simulink model "comparasion"  (R2023a)
settings: Solver=VariableStepAuto  StartTime=0.0  StopTime=3  RelTol=1e-3
values from neighbouring files (symbols this model uses):
  A = [a11 a21 a12 a22]    [calc_A.m]    (also in modelo.m = [a11 a12)
  Ad = [-1/t_beta 0 ... (first row only)    [calc_KMax.m]    (also in calc_Kmin.m; modelo.m)
  B = [b11 b21 b12 b22]    [calc_B.m]    (also in calc_inv_B.m = [b11 b12; b21 b22]; modelo.m = [b11 b12)
  C = [1 0 ... (first row only)    [modelo.m]
  D = [0 0;0 0]    [modelo.m]
  E = [e1 e2]    [calc_E.m]    (also in modelo.m = [e1)
  Ed = [k_beta/t_beta ... (first row only)    [calc_KMax.m]    (also in calc_Kmin.m; modelo.m)
  k1 = L_1(A,B,B2,C3,D32,D31,lambda)    [modelo.m]
  k2 = H_2_gain(A,B,B2,C2,D22)    [modelo.m]
  kH2Hinf = H_2_H_inf(A,B,B2,C2,D22,C1,D12,D11,a,b)    [modelo.m]
  kinf = H_inf(A,B,B2,C1,D12,D11)    [modelo.m]
  kLQ = LQ(Cz,Dzu,A,B,0)    [modelo.m]
  kLQR = LQ_R(Cz,Dzu,A,B,alpha,theta,r)    [modelo.m]
  x0 = [0, 0]    [modelo.m]
undefined symbols (not defined in the file or in its folder): sigbuilder_block
settings Model: Creator=Ferna  LastModifiedBy=Ferna

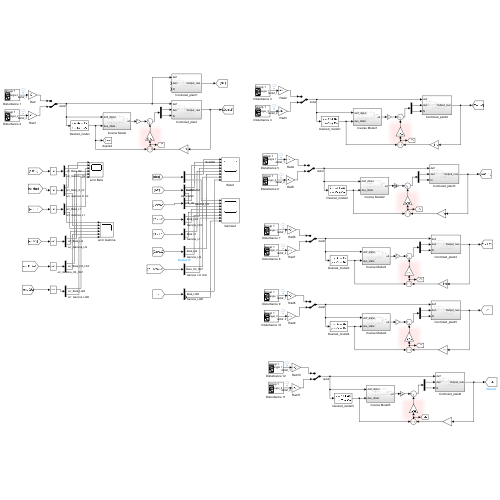
[thumbnail: Simulink's stored preview of the top-level diagram]
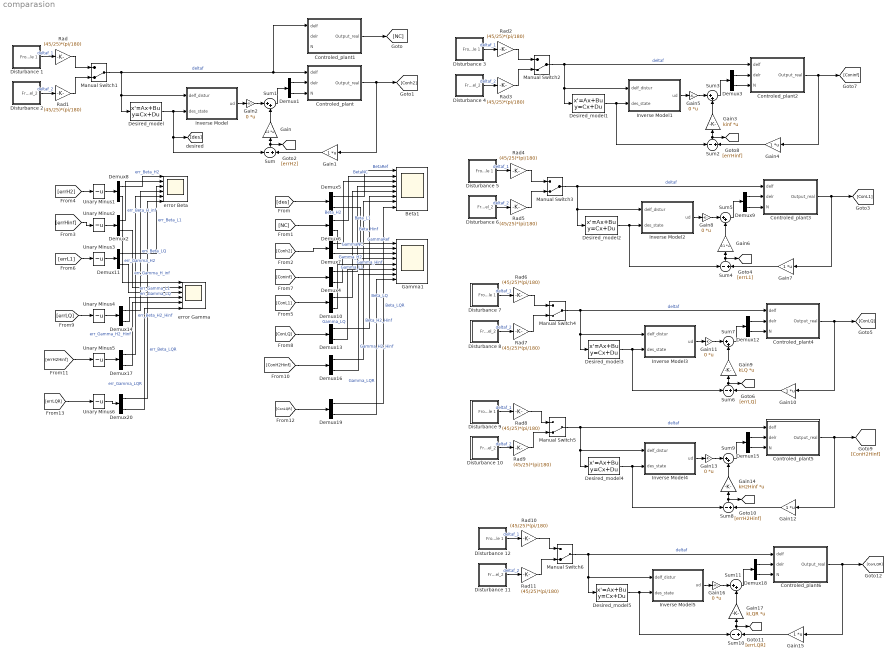
== system comparasion ==
  Beta1 : Scope  NumInputPorts=8
  Controled_plant : Subsystem
  Controled_plant1 : Subsystem
  Controled_plant2 : Subsystem
  Controled_plant3 : Subsystem
  Controled_plant4 : Subsystem
  Controled_plant5 : Subsystem
  Controled_plant6 : Subsystem
  Demux{1..20} (20 alike) : Demux  Outputs=2
  Desired_model{,1..5} (6 alike) : StateSpace  A=Ad  B=Ed  C=[1,0;0,1]  D=zeros(2,1)  InitialCondition=0
  Disturbance 1 : Subsystem  Tag=STV Subsys  LoadFcn=sigbuilder_block('load');  StartFcn=sigbuilder_block('start');  StopFcn=sigbuilder_block('stop');  ClipboardFcn=sigbuilder_block('clipboard');  mask(Sigbuilder block){tuvar=[0:10]}
      mask help: Simulink:masks:SigbuilderBlock_MD
      mask init:
      | if ~strcmp(get_param(bdroot(gcbh),'SimulationStatus'),'stopped') tuvar = sigbuilder_block('maskInit'); end
      settings: CopyFcn=sigbuilder_block('copy');  DeleteFcn=sigbuilder_block('delete');  ModelCloseFcn=sigbuilder_block('modelClose');  PreSaveFcn=sigbuilder_block('preSave');  PauseFcn=sigbuilder_block('pause');  ContinueFcn=sigbuilder_block('continue');  NameChangeFcn=sigbuilder_block('namechange');  OpenFcn=sigbuilder_block('open',[265.8 141.6 550.8 400.2 ]);  CloseFcn=sigbuilder_block('close');
      mask Display: plot(0, 0, 100, 100,[2, 2, 32, 32, 2], [68, 8, 8, 68, 68],[32, 2], [38, 38], [32, 19, 2],[53, 60, 44], [32, 17, 17, 2],[16, 16, 31, 31]);txt = getActiveGroup(gcbh);text(2, 100, txt,'verticalAlignment', 'top');
  Disturbance 10 : Subsystem  Tag=STV Subsys  LoadFcn=sigbuilder_block('load');  StartFcn=sigbuilder_block('start');  StopFcn=sigbuilder_block('stop');  ClipboardFcn=sigbuilder_block('clipboard');  mask(Sigbuilder block){tuvar=[0:10]}
      mask help: Simulink:masks:SigbuilderBlock_MD
      mask init:
      | if ~strcmp(get_param(bdroot(gcbh),'SimulationStatus'),'stopped') tuvar = sigbuilder_block('maskInit'); end
      settings: CopyFcn=sigbuilder_block('copy');  DeleteFcn=sigbuilder_block('delete');  ModelCloseFcn=sigbuilder_block('modelClose');  PreSaveFcn=sigbuilder_block('preSave');  PauseFcn=sigbuilder_block('pause');  ContinueFcn=sigbuilder_block('continue');  NameChangeFcn=sigbuilder_block('namechange');  OpenFcn=sigbuilder_block('open',[265.8 141.6 550.8 400.2 ]);  CloseFcn=sigbuilder_block('close');
      mask Display: plot(0, 0, 100, 100,[2, 2, 32, 32, 2], [68, 8, 8, 68, 68],[32, 2], [38, 38], [32, 19, 2],[53, 60, 44], [32, 17, 17, 2],[16, 16, 31, 31]);txt = getActiveGroup(gcbh);text(2, 100, txt,'verticalAlignment', 'top');
  Disturbance 11 : Subsystem  Tag=STV Subsys  LoadFcn=sigbuilder_block('load');  StartFcn=sigbuilder_block('start');  StopFcn=sigbuilder_block('stop');  ClipboardFcn=sigbuilder_block('clipboard');  mask(Sigbuilder block){tuvar=[0:10]}
      mask help: Simulink:masks:SigbuilderBlock_MD
      mask init:
      | if ~strcmp(get_param(bdroot(gcbh),'SimulationStatus'),'stopped') tuvar = sigbuilder_block('maskInit'); end
      settings: CopyFcn=sigbuilder_block('copy');  DeleteFcn=sigbuilder_block('delete');  ModelCloseFcn=sigbuilder_block('modelClose');  PreSaveFcn=sigbuilder_block('preSave');  PauseFcn=sigbuilder_block('pause');  ContinueFcn=sigbuilder_block('continue');  NameChangeFcn=sigbuilder_block('namechange');  OpenFcn=sigbuilder_block('open',[265.8 141.6 550.8 400.2 ]);  CloseFcn=sigbuilder_block('close');
      mask Display: plot(0, 0, 100, 100,[2, 2, 32, 32, 2], [68, 8, 8, 68, 68],[32, 2], [38, 38], [32, 19, 2],[53, 60, 44], [32, 17, 17, 2],[16, 16, 31, 31]);txt = getActiveGroup(gcbh);text(2, 100, txt,'verticalAlignment', 'top');
  Disturbance 12 : Subsystem  Tag=STV Subsys  LoadFcn=sigbuilder_block('load');  StartFcn=sigbuilder_block('start');  StopFcn=sigbuilder_block('stop');  ClipboardFcn=sigbuilder_block('clipboard');  mask(Sigbuilder block){tuvar=[0:10]}
      mask help: Simulink:masks:SigbuilderBlock_MD
      mask init:
      | if ~strcmp(get_param(bdroot(gcbh),'SimulationStatus'),'stopped') tuvar = sigbuilder_block('maskInit'); end
      settings: CopyFcn=sigbuilder_block('copy');  DeleteFcn=sigbuilder_block('delete');  ModelCloseFcn=sigbuilder_block('modelClose');  PreSaveFcn=sigbuilder_block('preSave');  PauseFcn=sigbuilder_block('pause');  ContinueFcn=sigbuilder_block('continue');  NameChangeFcn=sigbuilder_block('namechange');  OpenFcn=sigbuilder_block('open',[265.8 141.6 550.8 400.2 ]);  CloseFcn=sigbuilder_block('close');
      mask Display: plot(0, 0, 100, 100,[2, 2, 32, 32, 2], [68, 8, 8, 68, 68],[32, 2], [38, 38], [32, 19, 2],[53, 60, 44], [32, 17, 17, 2],[16, 16, 31, 31]);txt = getActiveGroup(gcbh);text(2, 100, txt,'verticalAlignment', 'top');
  Disturbance 2 : Subsystem  Tag=STV Subsys  LoadFcn=sigbuilder_block('load');  StartFcn=sigbuilder_block('start');  StopFcn=sigbuilder_block('stop');  ClipboardFcn=sigbuilder_block('clipboard');  mask(Sigbuilder block){tuvar=[0:10]}
      mask help: Simulink:masks:SigbuilderBlock_MD
      mask init:
      | if ~strcmp(get_param(bdroot(gcbh),'SimulationStatus'),'stopped') tuvar = sigbuilder_block('maskInit'); end
      settings: CopyFcn=sigbuilder_block('copy');  DeleteFcn=sigbuilder_block('delete');  ModelCloseFcn=sigbuilder_block('modelClose');  PreSaveFcn=sigbuilder_block('preSave');  PauseFcn=sigbuilder_block('pause');  ContinueFcn=sigbuilder_block('continue');  NameChangeFcn=sigbuilder_block('namechange');  OpenFcn=sigbuilder_block('open',[265.8 141.6 550.8 400.2 ]);  CloseFcn=sigbuilder_block('close');
      mask Display: plot(0, 0, 100, 100,[2, 2, 32, 32, 2], [68, 8, 8, 68, 68],[32, 2], [38, 38], [32, 19, 2],[53, 60, 44], [32, 17, 17, 2],[16, 16, 31, 31]);txt = getActiveGroup(gcbh);text(2, 100, txt,'verticalAlignment', 'top');
  Disturbance 3 : Subsystem  Tag=STV Subsys  LoadFcn=sigbuilder_block('load');  StartFcn=sigbuilder_block('start');  StopFcn=sigbuilder_block('stop');  ClipboardFcn=sigbuilder_block('clipboard');  mask(Sigbuilder block){tuvar=[0:10]}
      mask help: Simulink:masks:SigbuilderBlock_MD
      mask init:
      | if ~strcmp(get_param(bdroot(gcbh),'SimulationStatus'),'stopped') tuvar = sigbuilder_block('maskInit'); end
      settings: CopyFcn=sigbuilder_block('copy');  DeleteFcn=sigbuilder_block('delete');  ModelCloseFcn=sigbuilder_block('modelClose');  PreSaveFcn=sigbuilder_block('preSave');  PauseFcn=sigbuilder_block('pause');  ContinueFcn=sigbuilder_block('continue');  NameChangeFcn=sigbuilder_block('namechange');  OpenFcn=sigbuilder_block('open',[265.8 141.6 550.8 400.2 ]);  CloseFcn=sigbuilder_block('close');
      mask Display: plot(0, 0, 100, 100,[2, 2, 32, 32, 2], [68, 8, 8, 68, 68],[32, 2], [38, 38], [32, 19, 2],[53, 60, 44], [32, 17, 17, 2],[16, 16, 31, 31]);txt = getActiveGroup(gcbh);text(2, 100, txt,'verticalAlignment', 'top');
  Disturbance 4 : Subsystem  Tag=STV Subsys  LoadFcn=sigbuilder_block('load');  StartFcn=sigbuilder_block('start');  StopFcn=sigbuilder_block('stop');  ClipboardFcn=sigbuilder_block('clipboard');  mask(Sigbuilder block){tuvar=[0:10]}
      mask help: Simulink:masks:SigbuilderBlock_MD
      mask init:
      | if ~strcmp(get_param(bdroot(gcbh),'SimulationStatus'),'stopped') tuvar = sigbuilder_block('maskInit'); end
      settings: CopyFcn=sigbuilder_block('copy');  DeleteFcn=sigbuilder_block('delete');  ModelCloseFcn=sigbuilder_block('modelClose');  PreSaveFcn=sigbuilder_block('preSave');  PauseFcn=sigbuilder_block('pause');  ContinueFcn=sigbuilder_block('continue');  NameChangeFcn=sigbuilder_block('namechange');  OpenFcn=sigbuilder_block('open',[265.8 141.6 550.8 400.2 ]);  CloseFcn=sigbuilder_block('close');
      mask Display: plot(0, 0, 100, 100,[2, 2, 32, 32, 2], [68, 8, 8, 68, 68],[32, 2], [38, 38], [32, 19, 2],[53, 60, 44], [32, 17, 17, 2],[16, 16, 31, 31]);txt = getActiveGroup(gcbh);text(2, 100, txt,'verticalAlignment', 'top');
  Disturbance 5 : Subsystem  Tag=STV Subsys  LoadFcn=sigbuilder_block('load');  StartFcn=sigbuilder_block('start');  StopFcn=sigbuilder_block('stop');  ClipboardFcn=sigbuilder_block('clipboard');  mask(Sigbuilder block){tuvar=[0:10]}
      mask help: Simulink:masks:SigbuilderBlock_MD
      mask init:
      | if ~strcmp(get_param(bdroot(gcbh),'SimulationStatus'),'stopped') tuvar = sigbuilder_block('maskInit'); end
      settings: CopyFcn=sigbuilder_block('copy');  DeleteFcn=sigbuilder_block('delete');  ModelCloseFcn=sigbuilder_block('modelClose');  PreSaveFcn=sigbuilder_block('preSave');  PauseFcn=sigbuilder_block('pause');  ContinueFcn=sigbuilder_block('continue');  NameChangeFcn=sigbuilder_block('namechange');  OpenFcn=sigbuilder_block('open',[265.8 141.6 550.8 400.2 ]);  CloseFcn=sigbuilder_block('close');
      mask Display: plot(0, 0, 100, 100,[2, 2, 32, 32, 2], [68, 8, 8, 68, 68],[32, 2], [38, 38], [32, 19, 2],[53, 60, 44], [32, 17, 17, 2],[16, 16, 31, 31]);txt = getActiveGroup(gcbh);text(2, 100, txt,'verticalAlignment', 'top');
  Disturbance 6 : Subsystem  Tag=STV Subsys  LoadFcn=sigbuilder_block('load');  StartFcn=sigbuilder_block('start');  StopFcn=sigbuilder_block('stop');  ClipboardFcn=sigbuilder_block('clipboard');  mask(Sigbuilder block){tuvar=[0:10]}
      mask help: Simulink:masks:SigbuilderBlock_MD
      mask init:
      | if ~strcmp(get_param(bdroot(gcbh),'SimulationStatus'),'stopped') tuvar = sigbuilder_block('maskInit'); end
      settings: CopyFcn=sigbuilder_block('copy');  DeleteFcn=sigbuilder_block('delete');  ModelCloseFcn=sigbuilder_block('modelClose');  PreSaveFcn=sigbuilder_block('preSave');  PauseFcn=sigbuilder_block('pause');  ContinueFcn=sigbuilder_block('continue');  NameChangeFcn=sigbuilder_block('namechange');  OpenFcn=sigbuilder_block('open',[265.8 141.6 550.8 400.2 ]);  CloseFcn=sigbuilder_block('close');
      mask Display: plot(0, 0, 100, 100,[2, 2, 32, 32, 2], [68, 8, 8, 68, 68],[32, 2], [38, 38], [32, 19, 2],[53, 60, 44], [32, 17, 17, 2],[16, 16, 31, 31]);txt = getActiveGroup(gcbh);text(2, 100, txt,'verticalAlignment', 'top');
  Disturbance 7 : Subsystem  Tag=STV Subsys  LoadFcn=sigbuilder_block('load');  StartFcn=sigbuilder_block('start');  StopFcn=sigbuilder_block('stop');  ClipboardFcn=sigbuilder_block('clipboard');  mask(Sigbuilder block){tuvar=[0:10]}
      mask help: Simulink:masks:SigbuilderBlock_MD
      mask init:
      | if ~strcmp(get_param(bdroot(gcbh),'SimulationStatus'),'stopped') tuvar = sigbuilder_block('maskInit'); end
      settings: CopyFcn=sigbuilder_block('copy');  DeleteFcn=sigbuilder_block('delete');  ModelCloseFcn=sigbuilder_block('modelClose');  PreSaveFcn=sigbuilder_block('preSave');  PauseFcn=sigbuilder_block('pause');  ContinueFcn=sigbuilder_block('continue');  NameChangeFcn=sigbuilder_block('namechange');  OpenFcn=sigbuilder_block('open',[265.8 141.6 550.8 400.2 ]);  CloseFcn=sigbuilder_block('close');
      mask Display: plot(0, 0, 100, 100,[2, 2, 32, 32, 2], [68, 8, 8, 68, 68],[32, 2], [38, 38], [32, 19, 2],[53, 60, 44], [32, 17, 17, 2],[16, 16, 31, 31]);txt = getActiveGroup(gcbh);text(2, 100, txt,'verticalAlignment', 'top');
  Disturbance 8 : Subsystem  Tag=STV Subsys  LoadFcn=sigbuilder_block('load');  StartFcn=sigbuilder_block('start');  StopFcn=sigbuilder_block('stop');  ClipboardFcn=sigbuilder_block('clipboard');  mask(Sigbuilder block){tuvar=[0:10]}
      mask help: Simulink:masks:SigbuilderBlock_MD
      mask init:
      | if ~strcmp(get_param(bdroot(gcbh),'SimulationStatus'),'stopped') tuvar = sigbuilder_block('maskInit'); end
      settings: CopyFcn=sigbuilder_block('copy');  DeleteFcn=sigbuilder_block('delete');  ModelCloseFcn=sigbuilder_block('modelClose');  PreSaveFcn=sigbuilder_block('preSave');  PauseFcn=sigbuilder_block('pause');  ContinueFcn=sigbuilder_block('continue');  NameChangeFcn=sigbuilder_block('namechange');  OpenFcn=sigbuilder_block('open',[265.8 141.6 550.8 400.2 ]);  CloseFcn=sigbuilder_block('close');
      mask Display: plot(0, 0, 100, 100,[2, 2, 32, 32, 2], [68, 8, 8, 68, 68],[32, 2], [38, 38], [32, 19, 2],[53, 60, 44], [32, 17, 17, 2],[16, 16, 31, 31]);txt = getActiveGroup(gcbh);text(2, 100, txt,'verticalAlignment', 'top');
  Disturbance 9 : Subsystem  Tag=STV Subsys  LoadFcn=sigbuilder_block('load');  StartFcn=sigbuilder_block('start');  StopFcn=sigbuilder_block('stop');  ClipboardFcn=sigbuilder_block('clipboard');  mask(Sigbuilder block){tuvar=[0:10]}
      mask help: Simulink:masks:SigbuilderBlock_MD
      mask init:
      | if ~strcmp(get_param(bdroot(gcbh),'SimulationStatus'),'stopped') tuvar = sigbuilder_block('maskInit'); end
      settings: CopyFcn=sigbuilder_block('copy');  DeleteFcn=sigbuilder_block('delete');  ModelCloseFcn=sigbuilder_block('modelClose');  PreSaveFcn=sigbuilder_block('preSave');  PauseFcn=sigbuilder_block('pause');  ContinueFcn=sigbuilder_block('continue');  NameChangeFcn=sigbuilder_block('namechange');  OpenFcn=sigbuilder_block('open',[265.8 141.6 550.8 400.2 ]);  CloseFcn=sigbuilder_block('close');
      mask Display: plot(0, 0, 100, 100,[2, 2, 32, 32, 2], [68, 8, 8, 68, 68],[32, 2], [38, 38], [32, 19, 2],[53, 60, 44], [32, 17, 17, 2],[16, 16, 31, 31]);txt = getActiveGroup(gcbh);text(2, 100, txt,'verticalAlignment', 'top');
  Gain : Gain  Gain=k2  Multiplication=Matrix(K*u)
  Gain{1,4,7,10,12,15} (6 alike) : Gain  Multiplication=Matrix(K*u)
  Gain{2,5,8,11,13,16} (6 alike) : Gain  Gain=0  Multiplication=Matrix(K*u)
  Gain14 : Gain  Gain=kH2Hinf  Multiplication=Matrix(K*u)
  Gain17 : Gain  Gain=kLQR  Multiplication=Matrix(K*u)
  Gain3 : Gain  Gain=kinf  Multiplication=Matrix(K*u)
  Gain6 : Gain  Gain=k1  Multiplication=Matrix(K*u)
  Gain9 : Gain  Gain=kLQ  Multiplication=Matrix(K*u)
  Gamma1 : Scope  NumInputPorts=8
  Inverse Model : Subsystem
  Inverse Model1 : Subsystem
  Inverse Model2 : Subsystem
  Inverse Model3 : Subsystem
  Inverse Model4 : Subsystem
  Inverse Model5 : Subsystem
  Manual Switch{1..6} (6 alike) : ManualSwitch  CurrentSetting=0
  Rad{,1..11} (12 alike) : Gain  Gain=(45/25)*(pi/180)
  Sum{,2,4,6,8,10} (6 alike) : Sum  Inputs=-|+
  Sum{1,3,5,7,9,11} (6 alike) : Sum  Inputs=|++
  Unary Minus{1..6} (6 alike) : UnaryMinus
  error Beta : Scope  NumInputPorts=6
  error Gamma : Scope  NumInputPorts=6
  wires:
  Sum/1 -> [errH2], Gain/1
  Gain1/1 -> Sum/2
  Gain2/1 -> Sum1/1
  Demux1/1 -> Controled_plant/2(delr)
  Inverse Model/1(ud) -> Gain2/1
  Rad/1 -> Manual Switch1/1
  Controled_plant/1(Output_real) -> Gain1/1, [Conh2]
  Disturbance 2/1(Front steering angel_2) -> Rad1/1  "deltaf_2"
  Desired_model/1 -> [des], Sum/1, Inverse Model/2(des_state)
  Gain/1 -> Sum1/2
  Controled_plant1/1(Output_real) -> [NC]
  Sum1/1 -> Demux1/1
  Disturbance 1/1(Front sterring angle 1) -> Rad/1  "deltaf_1"
  Demux1/2 -> Controled_plant/3(N)
  Manual Switch1/1 -> Controled_plant1/1(delf), Controled_plant/1(delf), Inverse Model/1(delf_distur), Desired_model/1  "deltaf"
  Rad1/1 -> Manual Switch1/2
  Demux6/2 -> Gamma1/2  "GammaNC"
  Demux5/2 -> Gamma1/1  "GammaRef"
  [NC] -> Demux6/1
  Demux6/1 -> Beta1/2  "BetaNC"
  Demux7/2 -> Gamma1/3  "Gamma_H2"
  Demux7/1 -> Beta1/3  "Beta_H2"
  [des] -> Demux5/1
  Demux5/1 -> Beta1/1  "BetaRef"
  Rad3/1 -> Manual Switch2/2
  Manual Switch2/1 -> Controled_plant2/1(delf), Inverse Model1/1(delf_distur), Desired_model1/1  "deltaf"
  Sum3/1 -> Demux3/1
  Gain3/1 -> Sum3/2
  Disturbance 4/1(Front steering angel_2) -> Rad3/1  "deltaf_2"
  Desired_model1/1 -> Sum2/1, Inverse Model1/2(des_state)
  Controled_plant2/1(Output_real) -> Gain4/1, [Coninf]
  Inverse Model1/1(ud) -> Gain5/1
  Gain5/1 -> Sum3/1
  Rad2/1 -> Manual Switch2/1
  Demux3/1 -> Controled_plant2/2(delr)
  Gain4/1 -> Sum2/2
  Sum2/1 -> [errHinf], Gain3/1
  Demux3/2 -> Controled_plant2/3(N)
  Disturbance 3/1(Front sterring angle 1) -> Rad2/1  "deltaf_1"
  [Conh2] -> Demux7/1
  [Coninf] -> Demux4/1
  Demux4/1 -> Beta1/4  "Beta_Hinf"
  Demux4/2 -> Gamma1/4  "Gamma_Hinf"
  [errH2] -> Unary Minus1/1
  Unary Minus1/1 -> Demux8/1
  Demux8/1 -> error Beta/1  "err_Beta_H2"
  Demux8/2 -> error Gamma/1  "err_Gamma_H2"
  Demux2/1 -> error Beta/2  "err_Beta_H_inf"
  Demux2/2 -> error Gamma/2  "err_Gamma_H_inf"
  [errHinf] -> Unary Minus2/1
  Unary Minus2/1 -> Demux2/1
  Rad5/1 -> Manual Switch3/2
  Disturbance 5/1(Front sterring angle 1) -> Rad4/1  "deltaf_1"
  Manual Switch3/1 -> Controled_plant3/1(delf), Inverse Model2/1(delf_distur), Desired_model2/1  "deltaf"
  Sum5/1 -> Demux9/1
  Disturbance 6/1(Front steering angel_2) -> Rad5/1  "deltaf_2"
  Gain6/1 -> Sum5/2
  Gain7/1 -> Sum4/2
  Demux9/1 -> Controled_plant3/2(delr)
  Inverse Model2/1(ud) -> Gain8/1
  Rad4/1 -> Manual Switch3/1
  Gain8/1 -> Sum5/1
  Desired_model2/1 -> Sum4/1, Inverse Model2/2(des_state)
  Demux9/2 -> Controled_plant3/3(N)
  Sum4/1 -> [errL1], Gain6/1
  Controled_plant3/1(Output_real) -> Gain7/1, [ConL1]
  [ConL1] -> Demux10/1
  Demux10/1 -> Beta1/5  "Beta_L1"
  Demux10/2 -> Gamma1/5  "Gamma_L1"
  [errL1] -> Unary Minus3/1
  Unary Minus3/1 -> Demux11/1
  Demux11/1 -> error Beta/3  "err_Beta_L1"
  Demux11/2 -> error Gamma/3  "err_Gamma_L1"
  Controled_plant4/1(Output_real) -> [ConLQ], Gain10/1
  Sum6/1 -> Gain9/1, [errLQ]
  Demux12/2 -> Controled_plant4/3(N)
  Desired_model3/1 -> Inverse Model3/2(des_state), Sum6/1
  Gain11/1 -> Sum7/1
  Rad6/1 -> Manual Switch4/1
  Inverse Model3/1(ud) -> Gain11/1
  Demux12/1 -> Controled_plant4/2(delr)
  Gain10/1 -> Sum6/2
  Gain9/1 -> Sum7/2
  Disturbance 8/1(Front steering angel_2) -> Rad7/1  "deltaf_2"
  Sum7/1 -> Demux12/1
  Manual Switch4/1 -> Desired_model3/1, Inverse Model3/1(delf_distur), Controled_plant4/1(delf)  "deltaf"
  Disturbance 7/1(Front sterring angle 1) -> Rad6/1  "deltaf_1"
  Rad7/1 -> Manual Switch4/2
  [ConLQ] -> Demux13/1
  Demux13/1 -> Beta1/6  "Beta_LQ"
  Demux13/2 -> Gamma1/6  "Gamma_LQ"
  [errLQ] -> Unary Minus4/1
  Unary Minus4/1 -> Demux14/1
  Demux14/1 -> error Beta/4  "err_Beta_LQ"
  Demux14/2 -> error Gamma/4  "err_Gamma_LQ"
  Manual Switch5/1 -> Desired_model4/1, Inverse Model4/1(delf_distur), Controled_plant5/1(delf)  "deltaf"
  Rad8/1 -> Manual Switch5/1
  Desired_model4/1 -> Inverse Model4/2(des_state), Sum8/1
  Disturbance 9/1(Front sterring angle 1) -> Rad8/1  "deltaf_1"
  Demux15/1 -> Controled_plant5/2(delr)
  Inverse Model4/1(ud) -> Gain13/1
  Gain14/1 -> Sum9/2
  Sum9/1 -> Demux15/1
  Gain13/1 -> Sum9/1
  Disturbance 10/1(Front steering angel_2) -> Rad9/1  "deltaf_2"
  Rad9/1 -> Manual Switch5/2
  Gain12/1 -> Sum8/2
  Demux15/2 -> Controled_plant5/3(N)
  Controled_plant5/1(Output_real) -> [ConH2Hinf], Gain12/1
  Sum8/1 -> Gain14/1, [errH2Hinf]
  [ConH2Hinf] -> Demux16/1
  Demux16/1 -> Beta1/7  "Beta_H2_Hinf"
  Demux16/2 -> Gamma1/7  "Gamma_H2_Hinf"
  [errH2Hinf] -> Unary Minus5/1
  Demux17/1 -> error Beta/5  "err_Beta_H2_Hinf"
  Unary Minus5/1 -> Demux17/1
  Demux17/2 -> error Gamma/5  "err_Gamma_H2_Hinf"
  Sum10/1 -> [errLQR], Gain17/1
  Controled_plant6/1(Output_real) -> Gain15/1, [ConLQR]
  Demux18/2 -> Controled_plant6/3(N)
  Gain15/1 -> Sum10/2
  Rad11/1 -> Manual Switch6/2
  Disturbance 11/1(Front steering angel_2) -> Rad11/1  "deltaf_2"
  Gain16/1 -> Sum11/1
  Sum11/1 -> Demux18/1
  Gain17/1 -> Sum11/2
  Inverse Model5/1(ud) -> Gain16/1
  Demux18/1 -> Controled_plant6/2(delr)
  Disturbance 12/1(Front sterring angle 1) -> Rad10/1  "deltaf_1"
  Desired_model5/1 -> Sum10/1, Inverse Model5/2(des_state)
  Rad10/1 -> Manual Switch6/1
  Manual Switch6/1 -> Controled_plant6/1(delf), Inverse Model5/1(delf_distur), Desired_model5/1  "deltaf"
  [ConLQR] -> Demux19/1
  Demux19/1 -> Beta1/8  "Beta_LQR"
  Demux19/2 -> Gamma1/8  "Gamma_LQR"
  [errLQR] -> Unary Minus6/1
  Unary Minus6/1 -> Demux20/1
  Demux20/1 -> error Beta/6  "err_Beta_LQR"
  Demux20/2 -> error Gamma/6  "err_Gamma_LQR"

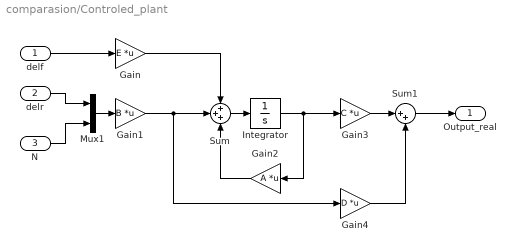
== system comparasion/Controled_plant ==
  delf : Inport
  delr : Inport  Port=2
  N : Inport  Port=3
  Gain : Gain  Gain=E  Multiplication=Matrix(K*u)
  Gain1 : Gain  Gain=B  Multiplication=Matrix(K*u)
  Gain2 : Gain  Gain=A  Multiplication=Matrix(K*u)
  Gain3 : Gain  Gain=C  Multiplication=Matrix(K*u)
  Gain4 : Gain  Gain=D  Multiplication=Matrix(K*u)
  Integrator : Integrator  InitialCondition=x0
  Mux1 : Mux  Inputs=2
  Sum : Sum  Inputs=+++
  Sum1 : Sum  Inputs=|++
  Output_real : Outport
  wires:
  Gain1/1 -> Gain4/1, Sum/2
  Gain4/1 -> Sum1/2
  delr/1 -> Mux1/1
  delf/1 -> Gain/1
  Integrator/1 -> Gain3/1, Gain2/1
  Gain/1 -> Sum/1
  Sum1/1 -> Output_real/1
  Gain3/1 -> Sum1/1
  N/1 -> Mux1/2
  Mux1/1 -> Gain1/1
  Sum/1 -> Integrator/1
  Gain2/1 -> Sum/3

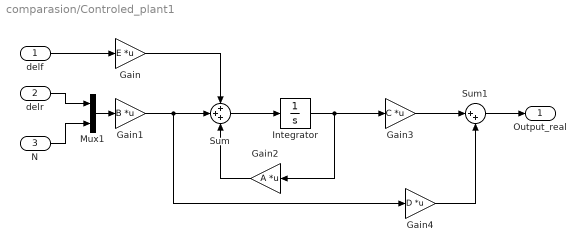
== system comparasion/Controled_plant1 ==
  delf : Inport
  delr : Inport  Port=2
  N : Inport  Port=3
  Gain : Gain  Gain=E  Multiplication=Matrix(K*u)
  Gain1 : Gain  Gain=B  Multiplication=Matrix(K*u)
  Gain2 : Gain  Gain=A  Multiplication=Matrix(K*u)
  Gain3 : Gain  Gain=C  Multiplication=Matrix(K*u)
  Gain4 : Gain  Gain=D  Multiplication=Matrix(K*u)
  Integrator : Integrator  InitialCondition=x0
  Mux1 : Mux  Inputs=2
  Sum : Sum  Inputs=+++
  Sum1 : Sum  Inputs=|++
  Output_real : Outport
  wires:
  Gain2/1 -> Sum/3
  Sum/1 -> Integrator/1
  Mux1/1 -> Gain1/1
  N/1 -> Mux1/2
  Gain3/1 -> Sum1/1
  Sum1/1 -> Output_real/1
  Gain/1 -> Sum/1
  Integrator/1 -> Gain2/1, Gain3/1
  delf/1 -> Gain/1
  delr/1 -> Mux1/1
  Gain4/1 -> Sum1/2
  Gain1/1 -> Sum/2, Gain4/1

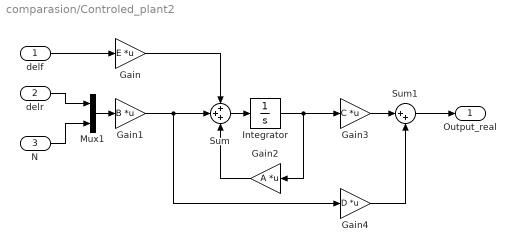
== system comparasion/Controled_plant2 ==
  delf : Inport
  delr : Inport  Port=2
  N : Inport  Port=3
  Gain : Gain  Gain=E  Multiplication=Matrix(K*u)
  Gain1 : Gain  Gain=B  Multiplication=Matrix(K*u)
  Gain2 : Gain  Gain=A  Multiplication=Matrix(K*u)
  Gain3 : Gain  Gain=C  Multiplication=Matrix(K*u)
  Gain4 : Gain  Gain=D  Multiplication=Matrix(K*u)
  Integrator : Integrator  InitialCondition=x0
  Mux1 : Mux  Inputs=2
  Sum : Sum  Inputs=+++
  Sum1 : Sum  Inputs=|++
  Output_real : Outport
  wires:
  Gain1/1 -> Gain4/1, Sum/2
  Gain4/1 -> Sum1/2
  delr/1 -> Mux1/1
  delf/1 -> Gain/1
  Integrator/1 -> Gain3/1, Gain2/1
  Gain/1 -> Sum/1
  Sum1/1 -> Output_real/1
  Gain3/1 -> Sum1/1
  N/1 -> Mux1/2
  Mux1/1 -> Gain1/1
  Sum/1 -> Integrator/1
  Gain2/1 -> Sum/3

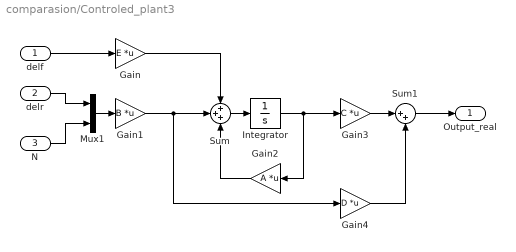
== system comparasion/Controled_plant3 ==
  delf : Inport
  delr : Inport  Port=2
  N : Inport  Port=3
  Gain : Gain  Gain=E  Multiplication=Matrix(K*u)
  Gain1 : Gain  Gain=B  Multiplication=Matrix(K*u)
  Gain2 : Gain  Gain=A  Multiplication=Matrix(K*u)
  Gain3 : Gain  Gain=C  Multiplication=Matrix(K*u)
  Gain4 : Gain  Gain=D  Multiplication=Matrix(K*u)
  Integrator : Integrator  InitialCondition=x0
  Mux1 : Mux  Inputs=2
  Sum : Sum  Inputs=+++
  Sum1 : Sum  Inputs=|++
  Output_real : Outport
  wires:
  Gain1/1 -> Gain4/1, Sum/2
  Gain4/1 -> Sum1/2
  delr/1 -> Mux1/1
  delf/1 -> Gain/1
  Integrator/1 -> Gain3/1, Gain2/1
  Gain/1 -> Sum/1
  Sum1/1 -> Output_real/1
  Gain3/1 -> Sum1/1
  N/1 -> Mux1/2
  Mux1/1 -> Gain1/1
  Sum/1 -> Integrator/1
  Gain2/1 -> Sum/3

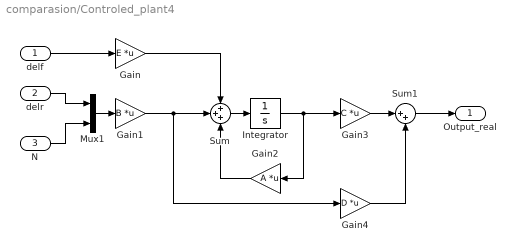
== system comparasion/Controled_plant4 ==
  delf : Inport
  delr : Inport  Port=2
  N : Inport  Port=3
  Gain : Gain  Gain=E  Multiplication=Matrix(K*u)
  Gain1 : Gain  Gain=B  Multiplication=Matrix(K*u)
  Gain2 : Gain  Gain=A  Multiplication=Matrix(K*u)
  Gain3 : Gain  Gain=C  Multiplication=Matrix(K*u)
  Gain4 : Gain  Gain=D  Multiplication=Matrix(K*u)
  Integrator : Integrator  InitialCondition=x0
  Mux1 : Mux  Inputs=2
  Sum : Sum  Inputs=+++
  Sum1 : Sum  Inputs=|++
  Output_real : Outport
  wires:
  Gain2/1 -> Sum/3
  Sum/1 -> Integrator/1
  Mux1/1 -> Gain1/1
  N/1 -> Mux1/2
  Gain3/1 -> Sum1/1
  Sum1/1 -> Output_real/1
  Gain/1 -> Sum/1
  Integrator/1 -> Gain2/1, Gain3/1
  delf/1 -> Gain/1
  delr/1 -> Mux1/1
  Gain4/1 -> Sum1/2
  Gain1/1 -> Sum/2, Gain4/1

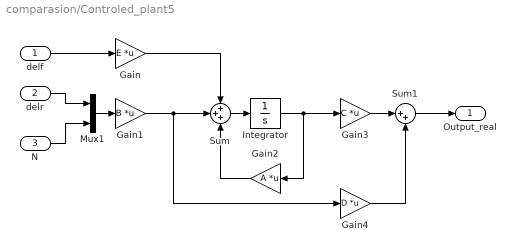
== system comparasion/Controled_plant5 ==
  delf : Inport
  delr : Inport  Port=2
  N : Inport  Port=3
  Gain : Gain  Gain=E  Multiplication=Matrix(K*u)
  Gain1 : Gain  Gain=B  Multiplication=Matrix(K*u)
  Gain2 : Gain  Gain=A  Multiplication=Matrix(K*u)
  Gain3 : Gain  Gain=C  Multiplication=Matrix(K*u)
  Gain4 : Gain  Gain=D  Multiplication=Matrix(K*u)
  Integrator : Integrator  InitialCondition=x0
  Mux1 : Mux  Inputs=2
  Sum : Sum  Inputs=+++
  Sum1 : Sum  Inputs=|++
  Output_real : Outport
  wires:
  Gain2/1 -> Sum/3
  Sum/1 -> Integrator/1
  Mux1/1 -> Gain1/1
  N/1 -> Mux1/2
  Gain3/1 -> Sum1/1
  Sum1/1 -> Output_real/1
  Gain/1 -> Sum/1
  Integrator/1 -> Gain2/1, Gain3/1
  delf/1 -> Gain/1
  delr/1 -> Mux1/1
  Gain4/1 -> Sum1/2
  Gain1/1 -> Sum/2, Gain4/1

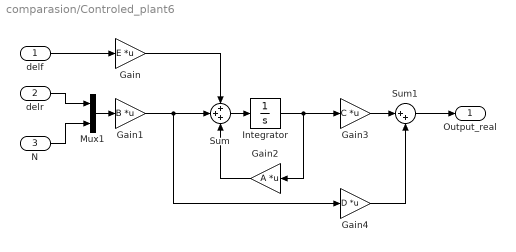
== system comparasion/Controled_plant6 ==
  delf : Inport
  delr : Inport  Port=2
  N : Inport  Port=3
  Gain : Gain  Gain=E  Multiplication=Matrix(K*u)
  Gain1 : Gain  Gain=B  Multiplication=Matrix(K*u)
  Gain2 : Gain  Gain=A  Multiplication=Matrix(K*u)
  Gain3 : Gain  Gain=C  Multiplication=Matrix(K*u)
  Gain4 : Gain  Gain=D  Multiplication=Matrix(K*u)
  Integrator : Integrator  InitialCondition=x0
  Mux1 : Mux  Inputs=2
  Sum : Sum  Inputs=+++
  Sum1 : Sum  Inputs=|++
  Output_real : Outport
  wires:
  Gain1/1 -> Gain4/1, Sum/2
  Gain4/1 -> Sum1/2
  delr/1 -> Mux1/1
  delf/1 -> Gain/1
  Integrator/1 -> Gain3/1, Gain2/1
  Gain/1 -> Sum/1
  Sum1/1 -> Output_real/1
  Gain3/1 -> Sum1/1
  N/1 -> Mux1/2
  Mux1/1 -> Gain1/1
  Sum/1 -> Integrator/1
  Gain2/1 -> Sum/3

== system comparasion/Disturbance 1 ==
  Demux : Demux  Tag=STV Demux  Outputs=1
      settings: DisplayOption=none
  FromWs : FromWorkspace  Tag=STV FromWs  VariableName=tuvar
      SigBuilderData=|
      | common.afterFinalStr = 'Extrapolate'
      | common.sampleTime = 0
      | dataSet.timeRange = [0 3]
      | dataSet.name = 'Group 1'
      | sbobj.Groups.Name = 'Group 1'
      | sbobj.Groups.Signals.Name = 'Front sterring angle 1'
      | sbobj.Groups.Signals.XData = [0 0.5 0.66 0.88 1.01 2.5 3]
      | sbobj.Groups.Signals.YData = [-0.01 0 0.2 0.8 1 1 1]
      | sbobj.Groups.TimeRange = [0 3]
  Front sterring angle 1 : Outport  Tag=STV Outport
  wires:
  FromWs/1 -> Demux/1
  Demux/1 -> Front sterring angle 1/1

== system comparasion/Disturbance 10 ==
  Demux : Demux  Tag=STV Demux  Outputs=1
      settings: DisplayOption=none
  FromWs : FromWorkspace  Tag=STV FromWs  VariableName=tuvar
      SigBuilderData=|
      | common.afterFinalStr = 'Extrapolate'
      | common.sampleTime = 0
      | dataSet.timeRange = [0 3]
      | dataSet.name = 'Group 1'
      | sbobj.Groups.Name = 'Group 1'
      | sbobj.Groups.Signals.Name = 'Front steering angel_2'
      | sbobj.Groups.Signals.XData = [0 0.187490625469 0.374981250937 0.562471876406 0.749962501875 0.937453127344 1.12494375281 1.31243437828 1.49992500375 1.68741562922 1.87490625469 2.06239688016 2.24988750562 2.43737813109 2.62486875656 2.81235938203 2.9998500075 3]
      | sbobj.Groups.Signals.YData = [0 0.565685424949 0.8 0.565685424949 9.79717439318e-17 -0.565685424949 -0.8 -0.565685424949 0 0 0 0 0 0 0 0 0 0]
      | sbobj.Groups.TimeRange = [0 3]
  Front steering angel_2 : Outport  Tag=STV Outport
  wires:
  FromWs/1 -> Demux/1
  Demux/1 -> Front steering angel_2/1

== system comparasion/Disturbance 11 ==
  Demux : Demux  Tag=STV Demux  Outputs=1
      settings: DisplayOption=none
  FromWs : FromWorkspace  Tag=STV FromWs  VariableName=tuvar
      SigBuilderData=|
      | common.afterFinalStr = 'Extrapolate'
      | common.sampleTime = 0
      | dataSet.timeRange = [0 3]
      | dataSet.name = 'Group 1'
      | sbobj.Groups.Name = 'Group 1'
      | sbobj.Groups.Signals.Name = 'Front steering angel_2'
      | sbobj.Groups.Signals.XData = [0 0.187490625469 0.374981250937 0.562471876406 0.749962501875 0.937453127344 1.12494375281 1.31243437828 1.49992500375 1.68741562922 1.87490625469 2.06239688016 2.24988750562 2.43737813109 2.62486875656 2.81235938203 2.9998500075 3]
      | sbobj.Groups.Signals.YData = [0 0.565685424949 0.8 0.565685424949 9.79717439318e-17 -0.565685424949 -0.8 -0.565685424949 0 0 0 0 0 0 0 0 0 0]
      | sbobj.Groups.TimeRange = [0 3]
  Front steering angel_2 : Outport  Tag=STV Outport
  wires:
  Demux/1 -> Front steering angel_2/1
  FromWs/1 -> Demux/1

== system comparasion/Disturbance 12 ==
  Demux : Demux  Tag=STV Demux  Outputs=1
      settings: DisplayOption=none
  FromWs : FromWorkspace  Tag=STV FromWs  VariableName=tuvar
      SigBuilderData=|
      | common.afterFinalStr = 'Extrapolate'
      | common.sampleTime = 0
      | dataSet.timeRange = [0 3]
      | dataSet.name = 'Group 1'
      | sbobj.Groups.Name = 'Group 1'
      | sbobj.Groups.Signals.Name = 'Front sterring angle 1'
      | sbobj.Groups.Signals.XData = [0 0.5 0.66 0.88 1.01 2.5 3]
      | sbobj.Groups.Signals.YData = [-0.01 0 0.2 0.8 1 1 1]
      | sbobj.Groups.TimeRange = [0 3]
  Front sterring angle 1 : Outport  Tag=STV Outport
  wires:
  FromWs/1 -> Demux/1
  Demux/1 -> Front sterring angle 1/1

== system comparasion/Disturbance 2 ==
  Demux : Demux  Tag=STV Demux  Outputs=1
      settings: DisplayOption=none
  FromWs : FromWorkspace  Tag=STV FromWs  VariableName=tuvar
      SigBuilderData=|
      | common.afterFinalStr = 'Extrapolate'
      | common.sampleTime = 0
      | dataSet.timeRange = [0 3]
      | dataSet.name = 'Group 1'
      | sbobj.Groups.Name = 'Group 1'
      | sbobj.Groups.Signals.Name = 'Front steering angel_2'
      | sbobj.Groups.Signals.XData = [0 0.187490625469 0.374981250937 0.562471876406 0.749962501875 0.937453127344 1.12494375281 1.31243437828 1.49992500375 1.68741562922 1.87490625469 2.06239688016 2.24988750562 2.43737813109 2.62486875656 2.81235938203 2.9998500075 3]
      | sbobj.Groups.Signals.YData = [0 0.565685424949 0.8 0.565685424949 9.79717439318e-17 -0.565685424949 -0.8 -0.565685424949 0 0 0 0 0 0 0 0 0 0]
      | sbobj.Groups.TimeRange = [0 3]
  Front steering angel_2 : Outport  Tag=STV Outport
  wires:
  Demux/1 -> Front steering angel_2/1
  FromWs/1 -> Demux/1

== system comparasion/Disturbance 3 ==
  Demux : Demux  Tag=STV Demux  Outputs=1
      settings: DisplayOption=none
  FromWs : FromWorkspace  Tag=STV FromWs  VariableName=tuvar
      SigBuilderData=|
      | common.afterFinalStr = 'Extrapolate'
      | common.sampleTime = 0
      | dataSet.timeRange = [0 3]
      | dataSet.name = 'Group 1'
      | sbobj.Groups.Name = 'Group 1'
      | sbobj.Groups.Signals.Name = 'Front sterring angle 1'
      | sbobj.Groups.Signals.XData = [0 0.5 0.66 0.88 1.01 2.5 3]
      | sbobj.Groups.Signals.YData = [-0.01 0 0.2 0.8 1 1 1]
      | sbobj.Groups.TimeRange = [0 3]
  Front sterring angle 1 : Outport  Tag=STV Outport
  wires:
  FromWs/1 -> Demux/1
  Demux/1 -> Front sterring angle 1/1

== system comparasion/Disturbance 4 ==
  Demux : Demux  Tag=STV Demux  Outputs=1
      settings: DisplayOption=none
  FromWs : FromWorkspace  Tag=STV FromWs  VariableName=tuvar
      SigBuilderData=|
      | common.afterFinalStr = 'Extrapolate'
      | common.sampleTime = 0
      | dataSet.timeRange = [0 3]
      | dataSet.name = 'Group 1'
      | sbobj.Groups.Name = 'Group 1'
      | sbobj.Groups.Signals.Name = 'Front steering angel_2'
      | sbobj.Groups.Signals.XData = [0 0.187490625469 0.374981250937 0.562471876406 0.749962501875 0.937453127344 1.12494375281 1.31243437828 1.49992500375 1.68741562922 1.87490625469 2.06239688016 2.24988750562 2.43737813109 2.62486875656 2.81235938203 2.9998500075 3]
      | sbobj.Groups.Signals.YData = [0 0.565685424949 0.8 0.565685424949 9.79717439318e-17 -0.565685424949 -0.8 -0.565685424949 0 0 0 0 0 0 0 0 0 0]
      | sbobj.Groups.TimeRange = [0 3]
  Front steering angel_2 : Outport  Tag=STV Outport
  wires:
  Demux/1 -> Front steering angel_2/1
  FromWs/1 -> Demux/1

== system comparasion/Disturbance 5 ==
  Demux : Demux  Tag=STV Demux  Outputs=1
      settings: DisplayOption=none
  FromWs : FromWorkspace  Tag=STV FromWs  VariableName=tuvar
      SigBuilderData=|
      | common.afterFinalStr = 'Extrapolate'
      | common.sampleTime = 0
      | dataSet.timeRange = [0 3]
      | dataSet.name = 'Group 1'
      | sbobj.Groups.Name = 'Group 1'
      | sbobj.Groups.Signals.Name = 'Front sterring angle 1'
      | sbobj.Groups.Signals.XData = [0 0.5 0.66 0.88 1.01 2.5 3]
      | sbobj.Groups.Signals.YData = [-0.01 0 0.2 0.8 1 1 1]
      | sbobj.Groups.TimeRange = [0 3]
  Front sterring angle 1 : Outport  Tag=STV Outport
  wires:
  FromWs/1 -> Demux/1
  Demux/1 -> Front sterring angle 1/1

== system comparasion/Disturbance 6 ==
  Demux : Demux  Tag=STV Demux  Outputs=1
      settings: DisplayOption=none
  FromWs : FromWorkspace  Tag=STV FromWs  VariableName=tuvar
      SigBuilderData=|
      | common.afterFinalStr = 'Extrapolate'
      | common.sampleTime = 0
      | dataSet.timeRange = [0 3]
      | dataSet.name = 'Group 1'
      | sbobj.Groups.Name = 'Group 1'
      | sbobj.Groups.Signals.Name = 'Front steering angel_2'
      | sbobj.Groups.Signals.XData = [0 0.187490625469 0.374981250937 0.562471876406 0.749962501875 0.937453127344 1.12494375281 1.31243437828 1.49992500375 1.68741562922 1.87490625469 2.06239688016 2.24988750562 2.43737813109 2.62486875656 2.81235938203 2.9998500075 3]
      | sbobj.Groups.Signals.YData = [0 0.565685424949 0.8 0.565685424949 9.79717439318e-17 -0.565685424949 -0.8 -0.565685424949 0 0 0 0 0 0 0 0 0 0]
      | sbobj.Groups.TimeRange = [0 3]
  Front steering angel_2 : Outport  Tag=STV Outport
  wires:
  Demux/1 -> Front steering angel_2/1
  FromWs/1 -> Demux/1

== system comparasion/Disturbance 7 ==
  Demux : Demux  Tag=STV Demux  Outputs=1
      settings: DisplayOption=none
  FromWs : FromWorkspace  Tag=STV FromWs  VariableName=tuvar
      SigBuilderData=|
      | common.afterFinalStr = 'Extrapolate'
      | common.sampleTime = 0
      | dataSet.timeRange = [0 3]
      | dataSet.name = 'Group 1'
      | sbobj.Groups.Name = 'Group 1'
      | sbobj.Groups.Signals.Name = 'Front sterring angle 1'
      | sbobj.Groups.Signals.XData = [0 0.5 0.66 0.88 1.01 2.5 3]
      | sbobj.Groups.Signals.YData = [-0.01 0 0.2 0.8 1 1 1]
      | sbobj.Groups.TimeRange = [0 3]
  Front sterring angle 1 : Outport  Tag=STV Outport
  wires:
  Demux/1 -> Front sterring angle 1/1
  FromWs/1 -> Demux/1

== system comparasion/Disturbance 8 ==
  Demux : Demux  Tag=STV Demux  Outputs=1
      settings: DisplayOption=none
  FromWs : FromWorkspace  Tag=STV FromWs  VariableName=tuvar
      SigBuilderData=|
      | common.afterFinalStr = 'Extrapolate'
      | common.sampleTime = 0
      | dataSet.timeRange = [0 3]
      | dataSet.name = 'Group 1'
      | sbobj.Groups.Name = 'Group 1'
      | sbobj.Groups.Signals.Name = 'Front steering angel_2'
      | sbobj.Groups.Signals.XData = [0 0.187490625469 0.374981250937 0.562471876406 0.749962501875 0.937453127344 1.12494375281 1.31243437828 1.49992500375 1.68741562922 1.87490625469 2.06239688016 2.24988750562 2.43737813109 2.62486875656 2.81235938203 2.9998500075 3]
      | sbobj.Groups.Signals.YData = [0 0.565685424949 0.8 0.565685424949 9.79717439318e-17 -0.565685424949 -0.8 -0.565685424949 0 0 0 0 0 0 0 0 0 0]
      | sbobj.Groups.TimeRange = [0 3]
  Front steering angel_2 : Outport  Tag=STV Outport
  wires:
  FromWs/1 -> Demux/1
  Demux/1 -> Front steering angel_2/1

== system comparasion/Disturbance 9 ==
  Demux : Demux  Tag=STV Demux  Outputs=1
      settings: DisplayOption=none
  FromWs : FromWorkspace  Tag=STV FromWs  VariableName=tuvar
      SigBuilderData=|
      | common.afterFinalStr = 'Extrapolate'
      | common.sampleTime = 0
      | dataSet.timeRange = [0 3]
      | dataSet.name = 'Group 1'
      | sbobj.Groups.Name = 'Group 1'
      | sbobj.Groups.Signals.Name = 'Front sterring angle 1'
      | sbobj.Groups.Signals.XData = [0 0.5 0.66 0.88 1.01 2.5 3]
      | sbobj.Groups.Signals.YData = [-0.01 0 0.2 0.8 1 1 1]
      | sbobj.Groups.TimeRange = [0 3]
  Front sterring angle 1 : Outport  Tag=STV Outport
  wires:
  Demux/1 -> Front sterring angle 1/1
  FromWs/1 -> Demux/1

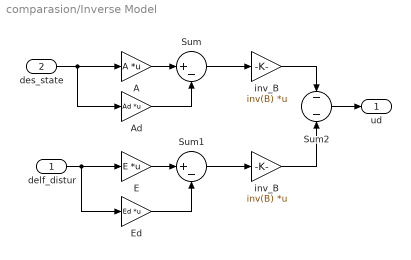
== system comparasion/Inverse Model ==
  delf_distur : Inport
  des_state : Inport  Port=2
  A : Gain  Gain=A  Multiplication=Matrix(K*u)
  Ad : Gain  Gain=Ad  Multiplication=Matrix(K*u)
  E : Gain  Gain=E  Multiplication=Matrix(K*u)
  Ed : Gain  Gain=Ed  Multiplication=Matrix(K*u)
  Sum : Sum  Inputs=|+-
  Sum1 : Sum  Inputs=|+-
  Sum2 : Sum  Inputs=-|-
  inv_B : Gain  Gain=inv(B)  Multiplication=Matrix(K*u)
  "inv_B " : Gain  Gain=inv(B)  Multiplication=Matrix(K*u)
  ud : Outport
  wires:
  E/1 -> Sum1/1
  Ad/1 -> Sum/2
  inv_B/1 -> Sum2/1
  delf_distur/1 -> Ed/1, E/1
  "inv_B "/1 -> Sum2/2
  Sum/1 -> inv_B/1
  A/1 -> Sum/1
  des_state/1 -> Ad/1, A/1
  Sum1/1 -> "inv_B "/1
  Sum2/1 -> ud/1
  Ed/1 -> Sum1/2

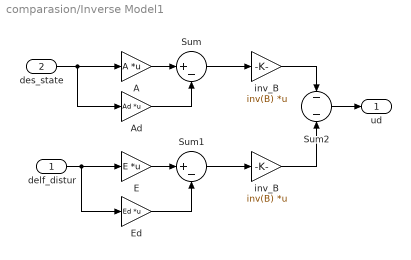
== system comparasion/Inverse Model1 ==
  delf_distur : Inport
  des_state : Inport  Port=2
  A : Gain  Gain=A  Multiplication=Matrix(K*u)
  Ad : Gain  Gain=Ad  Multiplication=Matrix(K*u)
  E : Gain  Gain=E  Multiplication=Matrix(K*u)
  Ed : Gain  Gain=Ed  Multiplication=Matrix(K*u)
  Sum : Sum  Inputs=|+-
  Sum1 : Sum  Inputs=|+-
  Sum2 : Sum  Inputs=-|-
  inv_B : Gain  Gain=inv(B)  Multiplication=Matrix(K*u)
  "inv_B " : Gain  Gain=inv(B)  Multiplication=Matrix(K*u)
  ud : Outport
  wires:
  E/1 -> Sum1/1
  Ad/1 -> Sum/2
  inv_B/1 -> Sum2/1
  delf_distur/1 -> Ed/1, E/1
  "inv_B "/1 -> Sum2/2
  Sum/1 -> inv_B/1
  A/1 -> Sum/1
  des_state/1 -> Ad/1, A/1
  Sum1/1 -> "inv_B "/1
  Sum2/1 -> ud/1
  Ed/1 -> Sum1/2

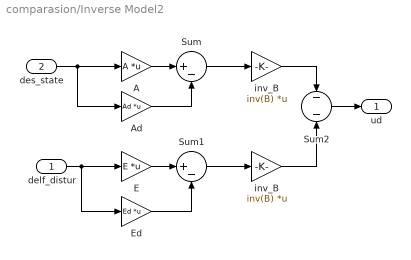
== system comparasion/Inverse Model2 ==
  delf_distur : Inport
  des_state : Inport  Port=2
  A : Gain  Gain=A  Multiplication=Matrix(K*u)
  Ad : Gain  Gain=Ad  Multiplication=Matrix(K*u)
  E : Gain  Gain=E  Multiplication=Matrix(K*u)
  Ed : Gain  Gain=Ed  Multiplication=Matrix(K*u)
  Sum : Sum  Inputs=|+-
  Sum1 : Sum  Inputs=|+-
  Sum2 : Sum  Inputs=-|-
  inv_B : Gain  Gain=inv(B)  Multiplication=Matrix(K*u)
  "inv_B " : Gain  Gain=inv(B)  Multiplication=Matrix(K*u)
  ud : Outport
  wires:
  E/1 -> Sum1/1
  Ad/1 -> Sum/2
  inv_B/1 -> Sum2/1
  delf_distur/1 -> Ed/1, E/1
  "inv_B "/1 -> Sum2/2
  Sum/1 -> inv_B/1
  A/1 -> Sum/1
  des_state/1 -> Ad/1, A/1
  Sum1/1 -> "inv_B "/1
  Sum2/1 -> ud/1
  Ed/1 -> Sum1/2

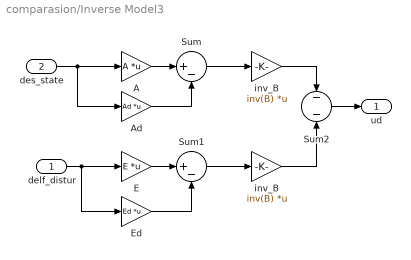
== system comparasion/Inverse Model3 ==
  delf_distur : Inport
  des_state : Inport  Port=2
  A : Gain  Gain=A  Multiplication=Matrix(K*u)
  Ad : Gain  Gain=Ad  Multiplication=Matrix(K*u)
  E : Gain  Gain=E  Multiplication=Matrix(K*u)
  Ed : Gain  Gain=Ed  Multiplication=Matrix(K*u)
  Sum : Sum  Inputs=|+-
  Sum1 : Sum  Inputs=|+-
  Sum2 : Sum  Inputs=-|-
  inv_B : Gain  Gain=inv(B)  Multiplication=Matrix(K*u)
  "inv_B " : Gain  Gain=inv(B)  Multiplication=Matrix(K*u)
  ud : Outport
  wires:
  Ed/1 -> Sum1/2
  Sum2/1 -> ud/1
  Sum1/1 -> "inv_B "/1
  des_state/1 -> A/1, Ad/1
  A/1 -> Sum/1
  Sum/1 -> inv_B/1
  "inv_B "/1 -> Sum2/2
  delf_distur/1 -> E/1, Ed/1
  inv_B/1 -> Sum2/1
  Ad/1 -> Sum/2
  E/1 -> Sum1/1

== system comparasion/Inverse Model4 ==
  delf_distur : Inport
  des_state : Inport  Port=2
  A : Gain  Gain=A  Multiplication=Matrix(K*u)
  Ad : Gain  Gain=Ad  Multiplication=Matrix(K*u)
  E : Gain  Gain=E  Multiplication=Matrix(K*u)
  Ed : Gain  Gain=Ed  Multiplication=Matrix(K*u)
  Sum : Sum  Inputs=|+-
  Sum1 : Sum  Inputs=|+-
  Sum2 : Sum  Inputs=-|-
  inv_B : Gain  Gain=inv(B)  Multiplication=Matrix(K*u)
  "inv_B " : Gain  Gain=inv(B)  Multiplication=Matrix(K*u)
  ud : Outport
  wires:
  Ed/1 -> Sum1/2
  Sum2/1 -> ud/1
  Sum1/1 -> "inv_B "/1
  des_state/1 -> A/1, Ad/1
  A/1 -> Sum/1
  Sum/1 -> inv_B/1
  "inv_B "/1 -> Sum2/2
  delf_distur/1 -> E/1, Ed/1
  inv_B/1 -> Sum2/1
  Ad/1 -> Sum/2
  E/1 -> Sum1/1

== system comparasion/Inverse Model5 ==
  delf_distur : Inport
  des_state : Inport  Port=2
  A : Gain  Gain=A  Multiplication=Matrix(K*u)
  Ad : Gain  Gain=Ad  Multiplication=Matrix(K*u)
  E : Gain  Gain=E  Multiplication=Matrix(K*u)
  Ed : Gain  Gain=Ed  Multiplication=Matrix(K*u)
  Sum : Sum  Inputs=|+-
  Sum1 : Sum  Inputs=|+-
  Sum2 : Sum  Inputs=-|-
  inv_B : Gain  Gain=inv(B)  Multiplication=Matrix(K*u)
  "inv_B " : Gain  Gain=inv(B)  Multiplication=Matrix(K*u)
  ud : Outport
  wires:
  E/1 -> Sum1/1
  Ad/1 -> Sum/2
  inv_B/1 -> Sum2/1
  delf_distur/1 -> Ed/1, E/1
  "inv_B "/1 -> Sum2/2
  Sum/1 -> inv_B/1
  A/1 -> Sum/1
  des_state/1 -> Ad/1, A/1
  Sum1/1 -> "inv_B "/1
  Sum2/1 -> ud/1
  Ed/1 -> Sum1/2
